simulink model "aufgabe_b1"  (R2016b)
settings: Solver=VariableStepAuto  StartTime=0.0  StopTime=10.0  RelTol=1e-3
settings Model: Creator=Thomas  LastModifiedBy=Thomas

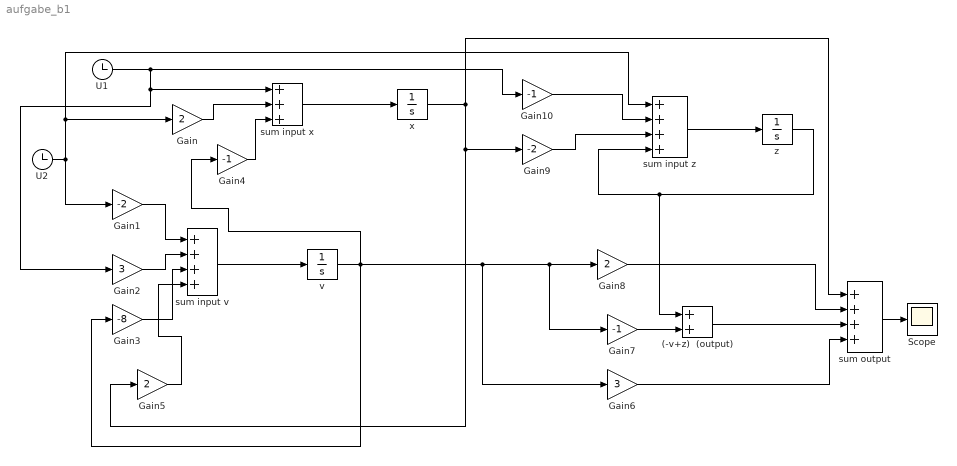
== system aufgabe_b1 ==
  (-v+z)  (output) : Sum
  Gain : Gain  Gain=2
  Gain1 : Gain  Gain=-2
  Gain10 : Gain  Gain=-1
  Gain2 : Gain  Gain=3
  Gain3 : Gain  Gain=-8
  Gain4 : Gain  Gain=-1
  Gain5 : Gain  Gain=2
  Gain6 : Gain  Gain=3
  Gain7 : Gain  Gain=-1
  Gain8 : Gain  Gain=2
  Gain9 : Gain  Gain=-2
  Scope : Scope
  U1 : Clock
  U2 : Clock
  sum input v : Sum  Inputs=++++
  sum input x : Sum  Inputs=+++
  sum input z : Sum  Inputs=++++
  sum output : Sum  Inputs=++++
  v : Integrator  InitialCondition=1
  x : Integrator  InitialCondition=1
  z : Integrator  InitialCondition=1
  wires:
  v/1 -> Gain3/1, Gain8/1, Gain7/1, Gain6/1, Gain4/1
  U2/1 -> Gain/1, sum input z/1, Gain1/1
  U1/1 -> Gain2/1, sum input x/1, Gain10/1
  x/1 -> Gain5/1, Gain9/1, sum output/1
  Gain5/1 -> sum input v/4
  sum input v/1 -> v/1
  sum input z/1 -> z/1
  z/1 -> sum input z/4, (-v+z)  (output)/1
  sum output/1 -> Scope/1
  (-v+z)  (output)/1 -> sum output/3
  Gain/1 -> sum input x/2
  Gain1/1 -> sum input v/1
  Gain2/1 -> sum input v/2
  Gain3/1 -> sum input v/3
  Gain4/1 -> sum input x/3
  Gain6/1 -> sum output/4
  Gain7/1 -> (-v+z)  (output)/2
  Gain8/1 -> sum output/2
  Gain9/1 -> sum input z/3
  sum input x/1 -> x/1
  Gain10/1 -> sum input z/2
